simulink model "fig2_52_simulink"  (R2021b)
settings: Solver=ode45  StartTime=0.0  StopTime=30  RelTol=1e-3  EnableMultiTasking=on
settings Model: Creator=One Informatic  LastModifiedBy=One Informatic
settings SolverCC: AlgebraicLoopSolver=TrustRegion
settings DataIOCC: LimitDataPoints=on  SaveFormat=Array  SignalLoggingSaveFormat=ModelDataLogs  ReturnWorkspaceOutputs=off
settings OptimizationCC: InitFltsAndDblsToZero=on  LifeSpan=inf
settings DebuggingCC: SaveWithParameterizedLinksMsg=none  UnderspecifiedInitializationDetection=Classic  MergeDetectMultiDrivingBlocksExec=none  SignalResolutionControl=TryResolveAllWithWarning  SolverPrmCheckMsg=warning  MultiTaskDSMMsg=warning  MultiTaskCondExecSysMsg=none  FcnCallInpInsideContextMsg=warning  SFUnexpectedBacktrackingDiag=warning  SFNoUnconditionalDefaultTransitionDiag=warning  SFExecutionAtInitializationDiag=none  SFMachineParentedDataDiag=warning  ArithmeticOperatorsInVariantConditions=warning
settings HardwareCC: ProdBitPerPointer=32  ProdBitPerSizeT=32  ProdBitPerPtrDiffT=32  ProdLargestAtomicFloat=None  ProdIntDivRoundTo=Undefined  ProdEndianess=Unspecified  ProdWordSize=32  ProdHWDeviceType=32-bit Generic
settings ModelReferenceCC: PropagateSignalLabelsOutOfModel=off
settings CodeAppCC: StateflowObjectComments=on
settings GRTTargetCC: TargetFcnLib=ansi_tfl_tmw.mat  TargetLangStandard=C89/C90 (ANSI)  CombineOutputUpdateFcns=off  GRTInterface=on
settings ConfigComp: CovMetricSettings=dw  CovSaveCumulativeToWorkspaceVar=on  CovSaveSingleToWorkspaceVar=on

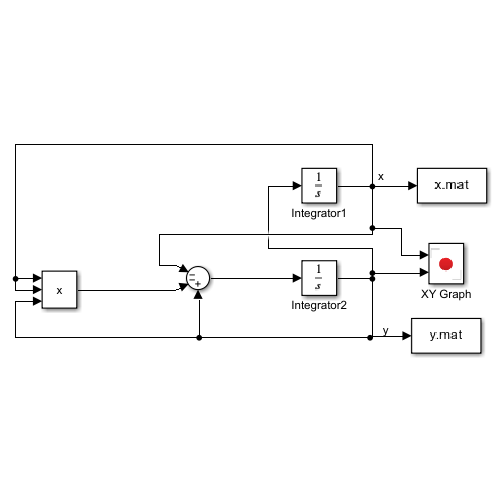
[thumbnail: Simulink's stored preview of the top-level diagram]
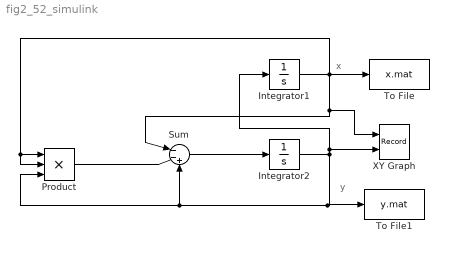
== system fig2_52_simulink ==
  note: y
  note: x
  Integrator1 : Integrator  InitialCondition=.1
  Integrator2 : Integrator  InitialCondition=.5
  Product : Product  Inputs=3  RndMeth=Zero
  Sum : Sum  Inputs=|--+
  To File : ToFile  Filename=x.mat  MatrixName=x  SampleTime=0.001
  To File1 : ToFile  Filename=y.mat  MatrixName=y  SampleTime=0.001
  XY Graph : Record  FileSettingsInternal="{\"entries\":[{\"content\":{\"excelSettings\":{\"content\":{},\"type\":\"Streamout.ExcelSettings\"}},\"type\":\"Streamout.FileSettingStorage\",\"uuid\":\"b89092a3-5b71-4315-a397-26b385c9cf46\"}],\"packageUris\":[\"http://schema.mathworks.com/mf0/streamout_blocks/R2020a\"],\"version\":\"1.0\"}"  Layout=[1 1]  SignalsInternal="{\"entries\":[{\"content\":{\"signals\":[{\"content\":{\"blockPath\":[\"CE4_3/XY Graph\"],\"channel\":[],\"dimensions\":[1],\"domain\":\"CE4_3/XY Graph\",\"lineColor\":\"#a2142f\",\"plots\":[1],\"port\":1,\"sid\":[],\"signalID\":283,\"signalName\":\"XY Graph:1\"},\"type\":\"RecordBlkView.Signal\",\"uuid\":\"8454dd79-2bde-4989-a44e-17789439d43f\"},{\"content\":{\"blockPath\":[\"CE4_3/XY Graph\"],\"channel\":[],\"dimensions\":[1],\"domain\":\"CE4_3/XY Graph\",\"lineColor\":\"#139fff\",\"plots\":[1],\"port\":2,\"sid\":[],\"signalID\":286,\"signalName\":\"XY Graph:2\"},\"type\":\"RecordBlkView.Signal\",\"uuid\":\"19130139-880e-492c-b6f9-84d5b3eed826\"}]},\"type\":\"RecordBlkView.InputSignals\",\"uuid\":\"9dafc7ad-6c8e-4d5d-940a-64217ea20ce9\"}],\"packageUris\":[\"http://schema.mathworks.com/mf0/streamout_blocks/R2020a\"],\"version\":\"1.0\"}"  VisualizationBindings="{\"xyplotplugin\":{\"info\":[{\"series\":[{\"bindingParametersList\":[{\"parameter\":\"X-Axis\",\"signalID\":283,\"signalName\":\"XY Graph:1\"},{\"parameter\":\"Y-Axis\",\"signalID\":286,\"signalName\":\"XY Graph:2\"}],\"seriesID\":23576}],\"subplotID\":1}]}}"  CompatibilityTag=XY  st=-1
  wires:
  Product/1 -> Sum/2
  Sum/1 -> Integrator2/1
  Integrator2/1 -> XY Graph/2, Integrator1/1, To File1/1, Product/3, Sum/3
  Integrator1/1 -> Sum/1, XY Graph/1, Product/2, Product/1, To File/1
